simulink model "model1"  (R2018b)
settings: Solver=ode4  StartTime=0.0  StopTime=6*R*C  FixedStep=1e-2  RelTol=1e-3
values from neighbouring files (symbols this model uses):
  K = 1/(R*C)    (= 1)    [Mikolaj_Ogarek_lab1.m]
  WPC = 0    [Mikolaj_Ogarek_lab1.m]
settings Model: Creator=mikolaj  LastModifiedBy=mikolaj

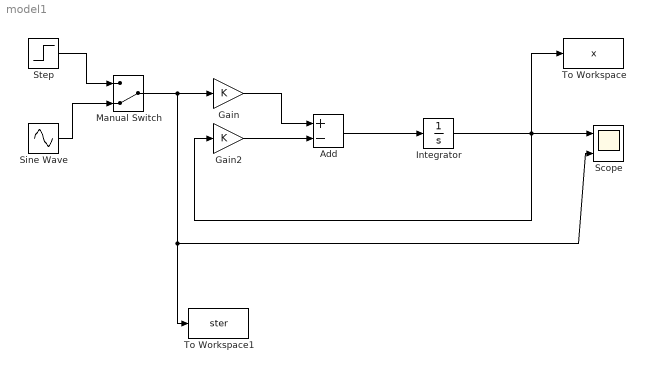
== system model1 ==
  Add : Sum  Inputs=+-
  Gain : Gain  Gain=K
  Gain2 : Gain  Gain=K
  Integrator : Integrator  InitialCondition=WPC
  Manual Switch : ManualSwitch  CurrentSetting=0
  Scope : Scope  NumInputPorts=2
  Sine Wave : Sin  Frequency=10  SampleTime=0
  Step : Step  Time=5  Before=3  After=0  SampleTime=0
  To Workspace : ToWorkspace  VariableName=x  SampleTime=-1
  To Workspace1 : ToWorkspace  VariableName=ster  SaveFormat=Timeseries  SampleTime=-1
  wires:
  Sine Wave/1 -> Manual Switch/2
  Gain/1 -> Add/1
  Add/1 -> Integrator/1
  Gain2/1 -> Add/2
  Integrator/1 -> Gain2/1, Scope/1, To Workspace/1
  Step/1 -> Manual Switch/1
  Manual Switch/1 -> To Workspace1/1, Scope/2, Gain/1
